simulink model "Control_test"  (R2014b)
settings: Solver=FixedStepDiscrete  StartTime=0.0  StopTime=Inf  FixedStep=0.001  RelTol=1e-3
PostLoadFcn:
  | , if any(exist('dsrtsu_mdlpostloadfcn', 'file') == [2, 3, 6]), try dsrtsu_mdlpostloadfcn('Execute', bdroot); catch fprintf('Error in PostLoadFcn (dsrtsu_mdlpostloadfcn) for model "%s":\n %s\n', bdroot, lasterr); end, end,
undefined symbols (not defined in the file or in its folder): dtLocal, slcm
libraries: rtican x163, simulink x14
(part 13 of 34)

== system Control_test/InputProcessing/CameraCanProcessing/Obstacle_Data_C_5 ==
  Bus Creator : BusCreator  Inputs=6
  Obstacle_Data_C_5 : rtican/RTICAN Receive (RX)   Reserved1=[]  Reserved2=[]  Reserved3=[]  Reserved4=[]  SfcnMessage=[]  Msg_Struct=[]  BoardTypeNo=[]  BoardNo=[]  ChannelNo=[]  Parameters=[]  DialogFcn=[]  UnitName=[]  Revision=[]  UnitValues=[]  DSProperties=struct('RTI',struct('Version',uint32(5),'BlockType',struct('isSLSource',uint8(1),'isSLSink',uint8(1),'isHWSource',uint8(0),'isHWSink',uint8(0),'isSetup',uint8(0),'isInline',uint8(1),'isNonInline',uint8(0),'isInterrupt',uint8(0),'isChannelwise',uint8(0)),'IOBoardType','RTICAN','UnitType','MESSAGE','Identifier','RX','DialogType','MSVC','BlockSet','RTICAN','SlaveProcessor','CAN'))  RTIBlockInterface=struct('OutputPortsWidth',int32([1 1 1 1 1 1]),'OutputPortsActive',[1 1 1 1 1 1],'OutputPortsName',{{'Alive_Counter_C_5','ObstacleWidth_C_5','ObjectMode_C_5','ObjectType_C_5','TTC_C_5','VisionScale_C_5'}},'OutputPortsDataType',{{'SS_DOUBLE','SS_DOUBLE','SS_DOUBLE','SS_DOUBLE','SS_DOUBLE','SS_DOUBLE'}},'OutputPortsLabel',{{'Alive_Counter_C_5','ObstacleWidth_C_5','ObjectMode_C_5','ObjectType_C_5','TTC_C_5','VisionScale_C_5'}},'OutputPortsLabelMode','ON','InputPortsWidth',int32(0),'InputPortsActive',0,'DialogFcn','rtican_message_interface_gui','BlockDisplay',{{'','center'}},'IconTransparency','on','ParameterTunableNames',{{}},'InitLevel',3,'BlockName',struct('Token',{{'Obstacle_Data_C_5'}}),'SampleTime',{{0.01}},'TriggerPort',{{'none'}},'EnablePort',{{'none'}})  RTIBlockParameters=struct('BoardTypeNo',{{1,'OFF',[]}},'BoardNo',{{1,'ON',[1 16]}},'ChannelNo',{{2,'ON',[1 2]}},'Parameters',{{struct('DataFileSupport',struct('DataFileSelectedMaster',1,'DataFileSelectedLocal',1,'DataFileName',['c:\users\mpc\desktop\hyundai car setup\rt2000_can_mod.dbc|c:\users\mpc\desktop\hyundai car setup\mobileye spec new\mobileye_mando_camera_ucb_v2.dbc|'],'DataFileDate',['18-Sep-2013 17:55:24'],'SelectedFile','..\..\dbcfiles\mobileye_mando_camera_ucb_v2.dbc','InterfaceFcn','rtican_dbc_file_parser'),'Options',struct('StatusSelected',0,'TimeSelected',0,'DeltaTimeSelected',0,'BytePortSelected',0,'MessageLengthSelected',0,'TriggerPort',struct('Selected',0,'TriggerType',0),'UserCoding',struct('Selected',0,'InterfaceFile','UserDecodingFile','FcnName','UserDecodeFcn','InportSelected',0,'InportWidth',1,'OutportSelected',0,'OutportWidth',1),'EnablePortSelected',0,'SignalOnPortnameSelected',1,'UseRXService',0),'Message',struct('MsgOnBlocknameSelected',1,'MsgName','Obstacle_Data_C_5','MsgIdFormat',0,'MsgId',1860,'MsgLength',6,'NumSignals',6,'SampleTime',0.01,'Signal',struct('SgnName',{'Alive_Counter_C_5','ObstacleWidth_C_5','ObjectMode_C_5','ObjectType_C_5','TTC_C_5','VisionScale_C_5'},'SgnStartBit',{0,8,16,18,22,32},'SgnLength',{2,8,2,4,10,12},'ByteLayout',{0,0,0,0,0,0},'Factor',{1,0.05,1,1,0.01,0.005},'Offset',{0,0,0,0,0,-8},'SgnComment',{'','','','','',''},'SgnUnit',{'','m','','','',''},'Min',{0,0,0,0,0,0},'Max',{0,0,0,0,0,0},'SgnType',{0,0,0,0,0,0},'SLDataType',{'SS_DOUBLE','SS_DOUBLE','SS_DOUBLE','SS_DOUBLE','SS_DOUBLE','SS_DOUBLE'},'DataType',{0,0,0,0,0,0},'ModeValue',{-1,-1,-1,-1,-1,-1}),'MsgIdNumFormat',0,'MsgComment',{{''}}),'Version',1.2,'general',struct('isFromLib',0)),'OFF',[]}},'GroupId',{{struct('Group',{{'RTICAN'}},'No',2,'Behavior',{{'NAMECHANGE'}},'BlockType',{{'SINK'}},'NameChangeFlag',0),'OFF',[]}},'SFcnRTICANMessage',{{struct('MsgType','RX','SFcnPortType','Scalar','MsgName','Obstacle_Data_C_5','MsgIdFormat','STD','MsgId',1860,'MsgLength',6,'NumSignals',6,'SampleTime',0.01,'Signal',struct('SgnName',{'Alive_Counter_C_5','ObstacleWidth_C_5','ObjectMode_C_5','ObjectType_C_5','TTC_C_5','VisionScale_C_5'},'SgnStartBit',{0,8,16,18,22,32},'SgnLength',{2,8,2,4,10,12},'ByteLayout',{['little endian'],['little endian'],['little endian'],['little endian'],['little endian'],['little endian']},'Factor',{1,0.05,1,1,0.01,0.005},'Offset',{0,0,0,0,0,-8},'SgnType',{'standard','standard','standard','standard','standard','standard'},'SLDataType',{'SS_DOUBLE','SS_DOUBLE','SS_DOUBLE','SS_DOUBLE','SS_DOUBLE','SS_DOUBLE'},'DataType',{['unsigned int'],['unsigned int'],['unsigned int'],['unsigned int'],['unsigned int'],['unsigned int']},'ModeValue',{-1,-1,-1,-1,-1,-1}),'StatusSelected','no','TimeSelected','no','DeltaTimeSelected','no','BytePortSelected','no','MessageLengthSelected','no','TriggerPort',struct('Selected','no','TriggerType',0),'UserCoding',struct('Selected','no','InterfaceFile','UserDecodingFile','FcnName','UserDecodeFcn','InportSelected','no','InportWidth',1,'OutportSelected','no','OutportWidth',1),'EnablePortSelected','no','UseRXService','no','BoardType','DS1','BoardNo',1,'ControllerNo',2),'OFF',[]}},'TLCFileName',{{'rtican_rx_message','OFF',[]}})  RTISFcnParameters=struct('SFcnRTICANMessage','struct','TLCFileName','char')  RTIBlockParaDefault=struct('BoardTypeNo',4302,'BoardNo',1,'ChannelNo',1,'Parameters',struct('DataFileSupport',struct('DataFileSelectedMaster',0,'DataFileSelectedLocal',0,'DataFileName','','DataFileDate','','SelectedFile',['<no file selected>']),'Options',struct('StatusSelected',1,'TimeSelected',1,'DeltaTimeSelected',1,'BytePortSelected',0,'MessageLengthSelected',0,'TriggerPort',struct('Selected',0,'TriggerType','rising'),'UserCoding',struct('Selected',0,'InterfaceFile','UserDecodingFile','FcnName','UserDecodeFcn','InportSelected',0,'InportWidth',1,'OutportSelected',0,'OutportWidth',1),'EnablePortSelected',0,'SignalOnPortnameSelected',1,'UseRXService',0),'Message',struct('MsgOnBlocknameSelected',0,'MsgName',['RX Message'],'MsgIdFormat',0,'MsgId',100,'MsgLength',8,'NumSignals',1,'SampleTime',-1,'Signal',struct('SgnName',['RX signal'],'SgnStartBit',0,'SgnLength',8,'SgnType',0,'ModeValue',-1,'DataType',0,'SLDataType','SS_DOUBLE','ByteLayout',0,'Factor',1,'Offset',0,'Min',0,'Max',255,'SgnComment',{{}},'SgnUnit',''),'MsgIdNumFormat',0,'MsgComment',{{''}}),'Version',1.2,'general',struct('isFromLib',1)),'GroupId',struct('Group',{{'RTICAN'}},'No',1,'Behavior',{{'NAMECHANGE'}},'BlockType',{{'SINK'}},'NameChangeFlag',0),'SFcnRTICANMessage',struct('MsgType','RX','MsgName',['RX Message'],'MsgIdFormat','STD','MsgId',100,'MsgLength',8,'NumSignals',1,'SampleTime',-1,'Signal',struct('SgnName',['RX signal'],'SgnStartBit',0,'SgnLength',8,'SgnType','standard','ModeValue',-1,'DataType',['unsigned int'],'ByteLayout',['little endian'],'SLDataType','SS_DOUBLE','Factor',1,'Offset',0),'StatusSelected','yes','TimeSelected','yes','DeltaTimeSelected','yes','BytePortSelected','no','MessageLengthSelected','no','EnablePortSelected','no','UserCoding',struct('Selected','no','InterfaceFile','UserDecodingFile','FcnName','UserDecodeFcn','InportSelected','no','InportWidth',1,'OutportSelected','no','OutportWidth',1),'TriggerPort',struct('Selected','no','TriggerType','rising'),'UseRXService','no','BoardType','DS4302','BoardNo',1,'ControllerNo',1,'SFcnPortType','Scalar'),'TLCFileName','rtican_rx_message')
      settings: AttributesFormatString=Group Id: RTICAN2\n
  Obstacle_Data_C_5_CAN : Outport
  wires:
  Bus Creator/1 -> Obstacle_Data_C_5_CAN/1
  Obstacle_Data_C_5/1 -> Bus Creator/1  "Alive_Counter_C_5"
  Obstacle_Data_C_5/2 -> Bus Creator/2  "ObstacleWidth_C_5"
  Obstacle_Data_C_5/3 -> Bus Creator/3  "ObjectMode_C_5"
  Obstacle_Data_C_5/4 -> Bus Creator/4  "ObjectType_C_5"
  Obstacle_Data_C_5/5 -> Bus Creator/5  "TTC_C_5"
  Obstacle_Data_C_5/6 -> Bus Creator/6  "VisionScale_C_5"

== system Control_test/InputProcessing/CameraCanProcessing/Obstacle_Data_C_6 ==
  Bus Creator : BusCreator  Inputs=6
  Obstacle_Data_C_6 : rtican/RTICAN Receive (RX)   Reserved1=[]  Reserved2=[]  Reserved3=[]  Reserved4=[]  SfcnMessage=[]  Msg_Struct=[]  BoardTypeNo=[]  BoardNo=[]  ChannelNo=[]  Parameters=[]  DialogFcn=[]  UnitName=[]  Revision=[]  UnitValues=[]  DSProperties=struct('RTI',struct('Version',uint32(5),'BlockType',struct('isSLSource',uint8(1),'isSLSink',uint8(1),'isHWSource',uint8(0),'isHWSink',uint8(0),'isSetup',uint8(0),'isInline',uint8(1),'isNonInline',uint8(0),'isInterrupt',uint8(0),'isChannelwise',uint8(0)),'IOBoardType','RTICAN','UnitType','MESSAGE','Identifier','RX','DialogType','MSVC','BlockSet','RTICAN','SlaveProcessor','CAN'))  RTIBlockInterface=struct('OutputPortsWidth',int32([1 1 1 1 1 1]),'OutputPortsActive',[1 1 1 1 1 1],'OutputPortsName',{{'Alive_Counter_C_6','ObstacleWidth_C_6','ObjectMode_C_6','ObjectType_C_6','TTC_C_6','VisionScale_C_6'}},'OutputPortsDataType',{{'SS_DOUBLE','SS_DOUBLE','SS_DOUBLE','SS_DOUBLE','SS_DOUBLE','SS_DOUBLE'}},'OutputPortsLabel',{{'Alive_Counter_C_6','ObstacleWidth_C_6','ObjectMode_C_6','ObjectType_C_6','TTC_C_6','VisionScale_C_6'}},'OutputPortsLabelMode','ON','InputPortsWidth',int32(0),'InputPortsActive',0,'DialogFcn','rtican_message_interface_gui','BlockDisplay',{{'','center'}},'IconTransparency','on','ParameterTunableNames',{{}},'InitLevel',3,'BlockName',struct('Token',{{'Obstacle_Data_C_6'}}),'SampleTime',{{0.01}},'TriggerPort',{{'none'}},'EnablePort',{{'none'}})  RTIBlockParameters=struct('BoardTypeNo',{{1,'OFF',[]}},'BoardNo',{{1,'ON',[1 16]}},'ChannelNo',{{2,'ON',[1 2]}},'Parameters',{{struct('DataFileSupport',struct('DataFileSelectedMaster',1,'DataFileSelectedLocal',1,'DataFileName',['c:\users\mpc\desktop\hyundai car setup\rt2000_can_mod.dbc|c:\users\mpc\desktop\hyundai car setup\mobileye spec new\mobileye_mando_camera_ucb_v2.dbc|'],'DataFileDate',['18-Sep-2013 17:55:24'],'SelectedFile','..\..\dbcfiles\mobileye_mando_camera_ucb_v2.dbc','InterfaceFcn','rtican_dbc_file_parser'),'Options',struct('StatusSelected',0,'TimeSelected',0,'DeltaTimeSelected',0,'BytePortSelected',0,'MessageLengthSelected',0,'TriggerPort',struct('Selected',0,'TriggerType',0),'UserCoding',struct('Selected',0,'InterfaceFile','UserDecodingFile','FcnName','UserDecodeFcn','InportSelected',0,'InportWidth',1,'OutportSelected',0,'OutportWidth',1),'EnablePortSelected',0,'SignalOnPortnameSelected',1,'UseRXService',0),'Message',struct('MsgOnBlocknameSelected',1,'MsgName','Obstacle_Data_C_6','MsgIdFormat',0,'MsgId',1863,'MsgLength',6,'NumSignals',6,'SampleTime',0.01,'Signal',struct('SgnName',{'Alive_Counter_C_6','ObstacleWidth_C_6','ObjectMode_C_6','ObjectType_C_6','TTC_C_6','VisionScale_C_6'},'SgnStartBit',{0,8,16,18,22,32},'SgnLength',{2,8,2,4,10,12},'ByteLayout',{0,0,0,0,0,0},'Factor',{1,0.05,1,1,0.01,0.005},'Offset',{0,0,0,0,0,-8},'SgnComment',{'','','','','',''},'SgnUnit',{'','m','','','',''},'Min',{0,0,0,0,0,0},'Max',{0,0,0,0,0,0},'SgnType',{0,0,0,0,0,0},'SLDataType',{'SS_DOUBLE','SS_DOUBLE','SS_DOUBLE','SS_DOUBLE','SS_DOUBLE','SS_DOUBLE'},'DataType',{0,0,0,0,0,0},'ModeValue',{-1,-1,-1,-1,-1,-1}),'MsgIdNumFormat',0,'MsgComment',{{''}}),'Version',1.2,'general',struct('isFromLib',0)),'OFF',[]}},'GroupId',{{struct('Group',{{'RTICAN'}},'No',2,'Behavior',{{'NAMECHANGE'}},'BlockType',{{'SINK'}},'NameChangeFlag',0),'OFF',[]}},'SFcnRTICANMessage',{{struct('MsgType','RX','SFcnPortType','Scalar','MsgName','Obstacle_Data_C_6','MsgIdFormat','STD','MsgId',1863,'MsgLength',6,'NumSignals',6,'SampleTime',0.01,'Signal',struct('SgnName',{'Alive_Counter_C_6','ObstacleWidth_C_6','ObjectMode_C_6','ObjectType_C_6','TTC_C_6','VisionScale_C_6'},'SgnStartBit',{0,8,16,18,22,32},'SgnLength',{2,8,2,4,10,12},'ByteLayout',{['little endian'],['little endian'],['little endian'],['little endian'],['little endian'],['little endian']},'Factor',{1,0.05,1,1,0.01,0.005},'Offset',{0,0,0,0,0,-8},'SgnType',{'standard','standard','standard','standard','standard','standard'},'SLDataType',{'SS_DOUBLE','SS_DOUBLE','SS_DOUBLE','SS_DOUBLE','SS_DOUBLE','SS_DOUBLE'},'DataType',{['unsigned int'],['unsigned int'],['unsigned int'],['unsigned int'],['unsigned int'],['unsigned int']},'ModeValue',{-1,-1,-1,-1,-1,-1}),'StatusSelected','no','TimeSelected','no','DeltaTimeSelected','no','BytePortSelected','no','MessageLengthSelected','no','TriggerPort',struct('Selected','no','TriggerType',0),'UserCoding',struct('Selected','no','InterfaceFile','UserDecodingFile','FcnName','UserDecodeFcn','InportSelected','no','InportWidth',1,'OutportSelected','no','OutportWidth',1),'EnablePortSelected','no','UseRXService','no','BoardType','DS1','BoardNo',1,'ControllerNo',2),'OFF',[]}},'TLCFileName',{{'rtican_rx_message','OFF',[]}})  RTISFcnParameters=struct('SFcnRTICANMessage','struct','TLCFileName','char')  RTIBlockParaDefault=struct('BoardTypeNo',4302,'BoardNo',1,'ChannelNo',1,'Parameters',struct('DataFileSupport',struct('DataFileSelectedMaster',0,'DataFileSelectedLocal',0,'DataFileName','','DataFileDate','','SelectedFile',['<no file selected>']),'Options',struct('StatusSelected',1,'TimeSelected',1,'DeltaTimeSelected',1,'BytePortSelected',0,'MessageLengthSelected',0,'TriggerPort',struct('Selected',0,'TriggerType','rising'),'UserCoding',struct('Selected',0,'InterfaceFile','UserDecodingFile','FcnName','UserDecodeFcn','InportSelected',0,'InportWidth',1,'OutportSelected',0,'OutportWidth',1),'EnablePortSelected',0,'SignalOnPortnameSelected',1,'UseRXService',0),'Message',struct('MsgOnBlocknameSelected',0,'MsgName',['RX Message'],'MsgIdFormat',0,'MsgId',100,'MsgLength',8,'NumSignals',1,'SampleTime',-1,'Signal',struct('SgnName',['RX signal'],'SgnStartBit',0,'SgnLength',8,'SgnType',0,'ModeValue',-1,'DataType',0,'SLDataType','SS_DOUBLE','ByteLayout',0,'Factor',1,'Offset',0,'Min',0,'Max',255,'SgnComment',{{}},'SgnUnit',''),'MsgIdNumFormat',0,'MsgComment',{{''}}),'Version',1.2,'general',struct('isFromLib',1)),'GroupId',struct('Group',{{'RTICAN'}},'No',1,'Behavior',{{'NAMECHANGE'}},'BlockType',{{'SINK'}},'NameChangeFlag',0),'SFcnRTICANMessage',struct('MsgType','RX','MsgName',['RX Message'],'MsgIdFormat','STD','MsgId',100,'MsgLength',8,'NumSignals',1,'SampleTime',-1,'Signal',struct('SgnName',['RX signal'],'SgnStartBit',0,'SgnLength',8,'SgnType','standard','ModeValue',-1,'DataType',['unsigned int'],'ByteLayout',['little endian'],'SLDataType','SS_DOUBLE','Factor',1,'Offset',0),'StatusSelected','yes','TimeSelected','yes','DeltaTimeSelected','yes','BytePortSelected','no','MessageLengthSelected','no','EnablePortSelected','no','UserCoding',struct('Selected','no','InterfaceFile','UserDecodingFile','FcnName','UserDecodeFcn','InportSelected','no','InportWidth',1,'OutportSelected','no','OutportWidth',1),'TriggerPort',struct('Selected','no','TriggerType','rising'),'UseRXService','no','BoardType','DS4302','BoardNo',1,'ControllerNo',1,'SFcnPortType','Scalar'),'TLCFileName','rtican_rx_message')
      settings: AttributesFormatString=Group Id: RTICAN2\n
  Obstacle_Data_C_6_CAN : Outport
  wires:
  Bus Creator/1 -> Obstacle_Data_C_6_CAN/1
  Obstacle_Data_C_6/1 -> Bus Creator/1  "Alive_Counter_C_6"
  Obstacle_Data_C_6/2 -> Bus Creator/2  "ObstacleWidth_C_6"
  Obstacle_Data_C_6/3 -> Bus Creator/3  "ObjectMode_C_6"
  Obstacle_Data_C_6/4 -> Bus Creator/4  "ObjectType_C_6"
  Obstacle_Data_C_6/5 -> Bus Creator/5  "TTC_C_6"
  Obstacle_Data_C_6/6 -> Bus Creator/6  "VisionScale_C_6"

== system Control_test/InputProcessing/CameraCanProcessing/Obstacle_Data_C_7 ==
  Bus Creator : BusCreator  Inputs=6
  Obstacle_Data_C_7 : rtican/RTICAN Receive (RX)   Reserved1=[]  Reserved2=[]  Reserved3=[]  Reserved4=[]  SfcnMessage=[]  Msg_Struct=[]  BoardTypeNo=[]  BoardNo=[]  ChannelNo=[]  Parameters=[]  DialogFcn=[]  UnitName=[]  Revision=[]  UnitValues=[]  DSProperties=struct('RTI',struct('Version',uint32(5),'BlockType',struct('isSLSource',uint8(1),'isSLSink',uint8(1),'isHWSource',uint8(0),'isHWSink',uint8(0),'isSetup',uint8(0),'isInline',uint8(1),'isNonInline',uint8(0),'isInterrupt',uint8(0),'isChannelwise',uint8(0)),'IOBoardType','RTICAN','UnitType','MESSAGE','Identifier','RX','DialogType','MSVC','BlockSet','RTICAN','SlaveProcessor','CAN'))  RTIBlockInterface=struct('OutputPortsWidth',int32([1 1 1 1 1 1]),'OutputPortsActive',[1 1 1 1 1 1],'OutputPortsName',{{'Alive_Counter_C_7','ObstacleWidth_C_7','ObjectMode_C_7','ObjectType_C_7','TTC_C_7','VisionScale_C_7'}},'OutputPortsDataType',{{'SS_DOUBLE','SS_DOUBLE','SS_DOUBLE','SS_DOUBLE','SS_DOUBLE','SS_DOUBLE'}},'OutputPortsLabel',{{'Alive_Counter_C_7','ObstacleWidth_C_7','ObjectMode_C_7','ObjectType_C_7','TTC_C_7','VisionScale_C_7'}},'OutputPortsLabelMode','ON','InputPortsWidth',int32(0),'InputPortsActive',0,'DialogFcn','rtican_message_interface_gui','BlockDisplay',{{'','center'}},'IconTransparency','on','ParameterTunableNames',{{}},'InitLevel',3,'BlockName',struct('Token',{{'Obstacle_Data_C_7'}}),'SampleTime',{{0.01}},'TriggerPort',{{'none'}},'EnablePort',{{'none'}})  RTIBlockParameters=struct('BoardTypeNo',{{1,'OFF',[]}},'BoardNo',{{1,'ON',[1 16]}},'ChannelNo',{{2,'ON',[1 2]}},'Parameters',{{struct('DataFileSupport',struct('DataFileSelectedMaster',1,'DataFileSelectedLocal',1,'DataFileName',['c:\users\mpc\desktop\hyundai car setup\rt2000_can_mod.dbc|c:\users\mpc\desktop\hyundai car setup\mobileye spec new\mobileye_mando_camera_ucb_v2.dbc|'],'DataFileDate',['18-Sep-2013 17:55:24'],'SelectedFile','..\..\dbcfiles\mobileye_mando_camera_ucb_v2.dbc','InterfaceFcn','rtican_dbc_file_parser'),'Options',struct('StatusSelected',0,'TimeSelected',0,'DeltaTimeSelected',0,'BytePortSelected',0,'MessageLengthSelected',0,'TriggerPort',struct('Selected',0,'TriggerType',0),'UserCoding',struct('Selected',0,'InterfaceFile','UserDecodingFile','FcnName','UserDecodeFcn','InportSelected',0,'InportWidth',1,'OutportSelected',0,'OutportWidth',1),'EnablePortSelected',0,'SignalOnPortnameSelected',1,'UseRXService',0),'Message',struct('MsgOnBlocknameSelected',1,'MsgName','Obstacle_Data_C_7','MsgIdFormat',0,'MsgId',1866,'MsgLength',6,'NumSignals',6,'SampleTime',0.01,'Signal',struct('SgnName',{'Alive_Counter_C_7','ObstacleWidth_C_7','ObjectMode_C_7','ObjectType_C_7','TTC_C_7','VisionScale_C_7'},'SgnStartBit',{0,8,16,18,22,32},'SgnLength',{2,8,2,4,10,12},'ByteLayout',{0,0,0,0,0,0},'Factor',{1,0.05,1,1,0.01,0.005},'Offset',{0,0,0,0,0,-8},'SgnComment',{'','','','','',''},'SgnUnit',{'','m','','','',''},'Min',{0,0,0,0,0,0},'Max',{0,0,0,0,0,0},'SgnType',{0,0,0,0,0,0},'SLDataType',{'SS_DOUBLE','SS_DOUBLE','SS_DOUBLE','SS_DOUBLE','SS_DOUBLE','SS_DOUBLE'},'DataType',{0,0,0,0,0,0},'ModeValue',{-1,-1,-1,-1,-1,-1}),'MsgIdNumFormat',0,'MsgComment',{{''}}),'Version',1.2,'general',struct('isFromLib',0)),'OFF',[]}},'GroupId',{{struct('Group',{{'RTICAN'}},'No',2,'Behavior',{{'NAMECHANGE'}},'BlockType',{{'SINK'}},'NameChangeFlag',0),'OFF',[]}},'SFcnRTICANMessage',{{struct('MsgType','RX','SFcnPortType','Scalar','MsgName','Obstacle_Data_C_7','MsgIdFormat','STD','MsgId',1866,'MsgLength',6,'NumSignals',6,'SampleTime',0.01,'Signal',struct('SgnName',{'Alive_Counter_C_7','ObstacleWidth_C_7','ObjectMode_C_7','ObjectType_C_7','TTC_C_7','VisionScale_C_7'},'SgnStartBit',{0,8,16,18,22,32},'SgnLength',{2,8,2,4,10,12},'ByteLayout',{['little endian'],['little endian'],['little endian'],['little endian'],['little endian'],['little endian']},'Factor',{1,0.05,1,1,0.01,0.005},'Offset',{0,0,0,0,0,-8},'SgnType',{'standard','standard','standard','standard','standard','standard'},'SLDataType',{'SS_DOUBLE','SS_DOUBLE','SS_DOUBLE','SS_DOUBLE','SS_DOUBLE','SS_DOUBLE'},'DataType',{['unsigned int'],['unsigned int'],['unsigned int'],['unsigned int'],['unsigned int'],['unsigned int']},'ModeValue',{-1,-1,-1,-1,-1,-1}),'StatusSelected','no','TimeSelected','no','DeltaTimeSelected','no','BytePortSelected','no','MessageLengthSelected','no','TriggerPort',struct('Selected','no','TriggerType',0),'UserCoding',struct('Selected','no','InterfaceFile','UserDecodingFile','FcnName','UserDecodeFcn','InportSelected','no','InportWidth',1,'OutportSelected','no','OutportWidth',1),'EnablePortSelected','no','UseRXService','no','BoardType','DS1','BoardNo',1,'ControllerNo',2),'OFF',[]}},'TLCFileName',{{'rtican_rx_message','OFF',[]}})  RTISFcnParameters=struct('SFcnRTICANMessage','struct','TLCFileName','char')  RTIBlockParaDefault=struct('BoardTypeNo',4302,'BoardNo',1,'ChannelNo',1,'Parameters',struct('DataFileSupport',struct('DataFileSelectedMaster',0,'DataFileSelectedLocal',0,'DataFileName','','DataFileDate','','SelectedFile',['<no file selected>']),'Options',struct('StatusSelected',1,'TimeSelected',1,'DeltaTimeSelected',1,'BytePortSelected',0,'MessageLengthSelected',0,'TriggerPort',struct('Selected',0,'TriggerType','rising'),'UserCoding',struct('Selected',0,'InterfaceFile','UserDecodingFile','FcnName','UserDecodeFcn','InportSelected',0,'InportWidth',1,'OutportSelected',0,'OutportWidth',1),'EnablePortSelected',0,'SignalOnPortnameSelected',1,'UseRXService',0),'Message',struct('MsgOnBlocknameSelected',0,'MsgName',['RX Message'],'MsgIdFormat',0,'MsgId',100,'MsgLength',8,'NumSignals',1,'SampleTime',-1,'Signal',struct('SgnName',['RX signal'],'SgnStartBit',0,'SgnLength',8,'SgnType',0,'ModeValue',-1,'DataType',0,'SLDataType','SS_DOUBLE','ByteLayout',0,'Factor',1,'Offset',0,'Min',0,'Max',255,'SgnComment',{{}},'SgnUnit',''),'MsgIdNumFormat',0,'MsgComment',{{''}}),'Version',1.2,'general',struct('isFromLib',1)),'GroupId',struct('Group',{{'RTICAN'}},'No',1,'Behavior',{{'NAMECHANGE'}},'BlockType',{{'SINK'}},'NameChangeFlag',0),'SFcnRTICANMessage',struct('MsgType','RX','MsgName',['RX Message'],'MsgIdFormat','STD','MsgId',100,'MsgLength',8,'NumSignals',1,'SampleTime',-1,'Signal',struct('SgnName',['RX signal'],'SgnStartBit',0,'SgnLength',8,'SgnType','standard','ModeValue',-1,'DataType',['unsigned int'],'ByteLayout',['little endian'],'SLDataType','SS_DOUBLE','Factor',1,'Offset',0),'StatusSelected','yes','TimeSelected','yes','DeltaTimeSelected','yes','BytePortSelected','no','MessageLengthSelected','no','EnablePortSelected','no','UserCoding',struct('Selected','no','InterfaceFile','UserDecodingFile','FcnName','UserDecodeFcn','InportSelected','no','InportWidth',1,'OutportSelected','no','OutportWidth',1),'TriggerPort',struct('Selected','no','TriggerType','rising'),'UseRXService','no','BoardType','DS4302','BoardNo',1,'ControllerNo',1,'SFcnPortType','Scalar'),'TLCFileName','rtican_rx_message')
      settings: AttributesFormatString=Group Id: RTICAN2\n
  Obstacle_Data_C_7_CAN : Outport
  wires:
  Bus Creator/1 -> Obstacle_Data_C_7_CAN/1
  Obstacle_Data_C_7/1 -> Bus Creator/1  "Alive_Counter_C_7"
  Obstacle_Data_C_7/2 -> Bus Creator/2  "ObstacleWidth_C_7"
  Obstacle_Data_C_7/3 -> Bus Creator/3  "ObjectMode_C_7"
  Obstacle_Data_C_7/4 -> Bus Creator/4  "ObjectType_C_7"
  Obstacle_Data_C_7/5 -> Bus Creator/5  "TTC_C_7"
  Obstacle_Data_C_7/6 -> Bus Creator/6  "VisionScale_C_7"

== system Control_test/InputProcessing/CameraCanProcessing/Obstacle_Data_C_8 ==
  Bus Creator : BusCreator  Inputs=6
  Obstacle_Data_C_8 : rtican/RTICAN Receive (RX)   Reserved1=[]  Reserved2=[]  Reserved3=[]  Reserved4=[]  SfcnMessage=[]  Msg_Struct=[]  BoardTypeNo=[]  BoardNo=[]  ChannelNo=[]  Parameters=[]  DialogFcn=[]  UnitName=[]  Revision=[]  UnitValues=[]  DSProperties=struct('RTI',struct('Version',uint32(5),'BlockType',struct('isSLSource',uint8(1),'isSLSink',uint8(1),'isHWSource',uint8(0),'isHWSink',uint8(0),'isSetup',uint8(0),'isInline',uint8(1),'isNonInline',uint8(0),'isInterrupt',uint8(0),'isChannelwise',uint8(0)),'IOBoardType','RTICAN','UnitType','MESSAGE','Identifier','RX','DialogType','MSVC','BlockSet','RTICAN','SlaveProcessor','CAN'))  RTIBlockInterface=struct('OutputPortsWidth',int32([1 1 1 1 1 1]),'OutputPortsActive',[1 1 1 1 1 1],'OutputPortsName',{{'Alive_Counter_C_8','ObstacleWidth_C_8','ObjectMode_C_8','ObjectType_C_8','TTC_C_8','VisionScale_C_8'}},'OutputPortsDataType',{{'SS_DOUBLE','SS_DOUBLE','SS_DOUBLE','SS_DOUBLE','SS_DOUBLE','SS_DOUBLE'}},'OutputPortsLabel',{{'Alive_Counter_C_8','ObstacleWidth_C_8','ObjectMode_C_8','ObjectType_C_8','TTC_C_8','VisionScale_C_8'}},'OutputPortsLabelMode','ON','InputPortsWidth',int32(0),'InputPortsActive',0,'DialogFcn','rtican_message_interface_gui','BlockDisplay',{{'','center'}},'IconTransparency','on','ParameterTunableNames',{{}},'InitLevel',3,'BlockName',struct('Token',{{'Obstacle_Data_C_8'}}),'SampleTime',{{0.01}},'TriggerPort',{{'none'}},'EnablePort',{{'none'}})  RTIBlockParameters=struct('BoardTypeNo',{{1,'OFF',[]}},'BoardNo',{{1,'ON',[1 16]}},'ChannelNo',{{2,'ON',[1 2]}},'Parameters',{{struct('DataFileSupport',struct('DataFileSelectedMaster',1,'DataFileSelectedLocal',1,'DataFileName',['c:\users\mpc\desktop\hyundai car setup\rt2000_can_mod.dbc|c:\users\mpc\desktop\hyundai car setup\mobileye spec new\mobileye_mando_camera_ucb_v2.dbc|'],'DataFileDate',['18-Sep-2013 17:55:24'],'SelectedFile','..\..\dbcfiles\mobileye_mando_camera_ucb_v2.dbc','InterfaceFcn','rtican_dbc_file_parser'),'Options',struct('StatusSelected',0,'TimeSelected',0,'DeltaTimeSelected',0,'BytePortSelected',0,'MessageLengthSelected',0,'TriggerPort',struct('Selected',0,'TriggerType',0),'UserCoding',struct('Selected',0,'InterfaceFile','UserDecodingFile','FcnName','UserDecodeFcn','InportSelected',0,'InportWidth',1,'OutportSelected',0,'OutportWidth',1),'EnablePortSelected',0,'SignalOnPortnameSelected',1,'UseRXService',0),'Message',struct('MsgOnBlocknameSelected',1,'MsgName','Obstacle_Data_C_8','MsgIdFormat',0,'MsgId',1869,'MsgLength',6,'NumSignals',6,'SampleTime',0.01,'Signal',struct('SgnName',{'Alive_Counter_C_8','ObstacleWidth_C_8','ObjectMode_C_8','ObjectType_C_8','TTC_C_8','VisionScale_C_8'},'SgnStartBit',{0,8,16,18,22,32},'SgnLength',{2,8,2,4,10,12},'ByteLayout',{0,0,0,0,0,0},'Factor',{1,0.05,1,1,0.01,0.005},'Offset',{0,0,0,0,0,-8},'SgnComment',{'','','','','',''},'SgnUnit',{'','m','','','',''},'Min',{0,0,0,0,0,0},'Max',{0,0,0,0,0,0},'SgnType',{0,0,0,0,0,0},'SLDataType',{'SS_DOUBLE','SS_DOUBLE','SS_DOUBLE','SS_DOUBLE','SS_DOUBLE','SS_DOUBLE'},'DataType',{0,0,0,0,0,0},'ModeValue',{-1,-1,-1,-1,-1,-1}),'MsgIdNumFormat',0,'MsgComment',{{''}}),'Version',1.2,'general',struct('isFromLib',0)),'OFF',[]}},'GroupId',{{struct('Group',{{'RTICAN'}},'No',2,'Behavior',{{'NAMECHANGE'}},'BlockType',{{'SINK'}},'NameChangeFlag',0),'OFF',[]}},'SFcnRTICANMessage',{{struct('MsgType','RX','SFcnPortType','Scalar','MsgName','Obstacle_Data_C_8','MsgIdFormat','STD','MsgId',1869,'MsgLength',6,'NumSignals',6,'SampleTime',0.01,'Signal',struct('SgnName',{'Alive_Counter_C_8','ObstacleWidth_C_8','ObjectMode_C_8','ObjectType_C_8','TTC_C_8','VisionScale_C_8'},'SgnStartBit',{0,8,16,18,22,32},'SgnLength',{2,8,2,4,10,12},'ByteLayout',{['little endian'],['little endian'],['little endian'],['little endian'],['little endian'],['little endian']},'Factor',{1,0.05,1,1,0.01,0.005},'Offset',{0,0,0,0,0,-8},'SgnType',{'standard','standard','standard','standard','standard','standard'},'SLDataType',{'SS_DOUBLE','SS_DOUBLE','SS_DOUBLE','SS_DOUBLE','SS_DOUBLE','SS_DOUBLE'},'DataType',{['unsigned int'],['unsigned int'],['unsigned int'],['unsigned int'],['unsigned int'],['unsigned int']},'ModeValue',{-1,-1,-1,-1,-1,-1}),'StatusSelected','no','TimeSelected','no','DeltaTimeSelected','no','BytePortSelected','no','MessageLengthSelected','no','TriggerPort',struct('Selected','no','TriggerType',0),'UserCoding',struct('Selected','no','InterfaceFile','UserDecodingFile','FcnName','UserDecodeFcn','InportSelected','no','InportWidth',1,'OutportSelected','no','OutportWidth',1),'EnablePortSelected','no','UseRXService','no','BoardType','DS1','BoardNo',1,'ControllerNo',2),'OFF',[]}},'TLCFileName',{{'rtican_rx_message','OFF',[]}})  RTISFcnParameters=struct('SFcnRTICANMessage','struct','TLCFileName','char')  RTIBlockParaDefault=struct('BoardTypeNo',4302,'BoardNo',1,'ChannelNo',1,'Parameters',struct('DataFileSupport',struct('DataFileSelectedMaster',0,'DataFileSelectedLocal',0,'DataFileName','','DataFileDate','','SelectedFile',['<no file selected>']),'Options',struct('StatusSelected',1,'TimeSelected',1,'DeltaTimeSelected',1,'BytePortSelected',0,'MessageLengthSelected',0,'TriggerPort',struct('Selected',0,'TriggerType','rising'),'UserCoding',struct('Selected',0,'InterfaceFile','UserDecodingFile','FcnName','UserDecodeFcn','InportSelected',0,'InportWidth',1,'OutportSelected',0,'OutportWidth',1),'EnablePortSelected',0,'SignalOnPortnameSelected',1,'UseRXService',0),'Message',struct('MsgOnBlocknameSelected',0,'MsgName',['RX Message'],'MsgIdFormat',0,'MsgId',100,'MsgLength',8,'NumSignals',1,'SampleTime',-1,'Signal',struct('SgnName',['RX signal'],'SgnStartBit',0,'SgnLength',8,'SgnType',0,'ModeValue',-1,'DataType',0,'SLDataType','SS_DOUBLE','ByteLayout',0,'Factor',1,'Offset',0,'Min',0,'Max',255,'SgnComment',{{}},'SgnUnit',''),'MsgIdNumFormat',0,'MsgComment',{{''}}),'Version',1.2,'general',struct('isFromLib',1)),'GroupId',struct('Group',{{'RTICAN'}},'No',1,'Behavior',{{'NAMECHANGE'}},'BlockType',{{'SINK'}},'NameChangeFlag',0),'SFcnRTICANMessage',struct('MsgType','RX','MsgName',['RX Message'],'MsgIdFormat','STD','MsgId',100,'MsgLength',8,'NumSignals',1,'SampleTime',-1,'Signal',struct('SgnName',['RX signal'],'SgnStartBit',0,'SgnLength',8,'SgnType','standard','ModeValue',-1,'DataType',['unsigned int'],'ByteLayout',['little endian'],'SLDataType','SS_DOUBLE','Factor',1,'Offset',0),'StatusSelected','yes','TimeSelected','yes','DeltaTimeSelected','yes','BytePortSelected','no','MessageLengthSelected','no','EnablePortSelected','no','UserCoding',struct('Selected','no','InterfaceFile','UserDecodingFile','FcnName','UserDecodeFcn','InportSelected','no','InportWidth',1,'OutportSelected','no','OutportWidth',1),'TriggerPort',struct('Selected','no','TriggerType','rising'),'UseRXService','no','BoardType','DS4302','BoardNo',1,'ControllerNo',1,'SFcnPortType','Scalar'),'TLCFileName','rtican_rx_message')
      settings: AttributesFormatString=Group Id: RTICAN2\n
  Obstacle_Data_C_8_CAN : Outport
  wires:
  Bus Creator/1 -> Obstacle_Data_C_8_CAN/1
  Obstacle_Data_C_8/1 -> Bus Creator/1  "Alive_Counter_C_8"
  Obstacle_Data_C_8/2 -> Bus Creator/2  "ObstacleWidth_C_8"
  Obstacle_Data_C_8/3 -> Bus Creator/3  "ObjectMode_C_8"
  Obstacle_Data_C_8/4 -> Bus Creator/4  "ObjectType_C_8"
  Obstacle_Data_C_8/5 -> Bus Creator/5  "TTC_C_8"
  Obstacle_Data_C_8/6 -> Bus Creator/6  "VisionScale_C_8"

== system Control_test/InputProcessing/IBEOCANProcessing/IBEOESP2Processing ==
  In1 : Inport
  Bus Creator : BusCreator  Inputs=12
  Bus Selector3 : BusSelector  OutputSignals=LAT_ACCEL,LAT_ACCEL_STAT,LAT_ACCEL_DIAG,LONG_ACCEL,LONG_ACCEL_STAT,LONG_ACCEL_DIAG,CYL_PRES,CYL_PRES_STAT,CYL_PRESS_DIAG,YAW_RATE,YAW_RATE_STAT,YAW_RATE_DIAG
  ESP2 Processing : Subsystem
  Out1 : Outport
  wires:
  Bus Selector3/1 -> ESP2 Processing/1(LAT_ACCEL_CAN)  "<LAT_ACCEL>"
  Bus Selector3/2 -> ESP2 Processing/2(LAT_ACCEL_STAT_CAN)  "<LAT_ACCEL_STAT>"
  Bus Selector3/3 -> ESP2 Processing/3(LAT_ACCEL_DIAG_CAN)  "<LAT_ACCEL_DIAG>"
  Bus Selector3/4 -> ESP2 Processing/4(LONG_ACCEL_CAN)  "<LONG_ACCEL>"
  Bus Selector3/5 -> ESP2 Processing/5(LONG_ACCEL_STAT_CAN)  "<LONG_ACCEL_STAT>"
  Bus Selector3/6 -> ESP2 Processing/6(LONG_ACCEL_DIAG_CAN)  "<LONG_ACCEL_DIAG>"
  Bus Selector3/7 -> ESP2 Processing/7(CYL_PRES_CAN)  "<CYL_PRES>"
  Bus Selector3/8 -> ESP2 Processing/8(CYL_PRES_STAT_CAN)  "<CYL_PRES_STAT>"
  Bus Selector3/9 -> ESP2 Processing/9(CYL_PRES_DIAG_CAN)  "<CYL_PRESS_DIAG>"
  Bus Selector3/10 -> ESP2 Processing/10(YAW_RATE_CAN)  "<YAW_RATE>"
  Bus Selector3/11 -> ESP2 Processing/11(YAW_RATE_STAT_CAN)  "<YAW_RATE_STAT>"
  Bus Selector3/12 -> ESP2 Processing/12(YAW_RATE_DIAG_CAN)  "<YAW_RATE_DIAG>"
  ESP2 Processing/1(ipLatAccel [m/s2]) -> Bus Creator/1
  ESP2 Processing/2(ipLatAccelFail) -> Bus Creator/2
  ESP2 Processing/3(ipLatAccelDiag) -> Bus Creator/3
  ESP2 Processing/4(ipLongAccel [m/s2]) -> Bus Creator/4
  ESP2 Processing/5(ipLongAccelFail) -> Bus Creator/5
  ESP2 Processing/6(ipLongAccelDiag) -> Bus Creator/6
  ESP2 Processing/7(ipMsCylPress [bar]) -> Bus Creator/7
  ESP2 Processing/8(ipMsCylPressFail) -> Bus Creator/8
  ESP2 Processing/9(ipMsCylPressDiag) -> Bus Creator/9
  ESP2 Processing/10(ipYawRate [deg/s]) -> Bus Creator/10
  ESP2 Processing/11(ipYawRateFail) -> Bus Creator/11
  ESP2 Processing/12(ipYawRateDiag) -> Bus Creator/12
  Bus Creator/1 -> Out1/1  "ESP2DataCAN3"
  In1/1 -> Bus Selector3/1

== system Control_test/InputProcessing/IBEOCANProcessing/IBEOSASProcessing ==
  In1 : Inport
  Bus Creator4 : BusCreator  Inputs=6
  Bus Selector4 : BusSelector  OutputSignals=SAS_Angle,SAS_Speed,MsgCount,CheckSum
  SAS1 Processing : Subsystem
  Out1 : Outport
  wires:
  Bus Selector4/1 -> SAS1 Processing/1(SAS_Angle_CAN)  "<SAS_Angle>"
  Bus Selector4/2 -> SAS1 Processing/2(SAS_Speed_CAN)  "<SAS_Speed>"
  Bus Selector4/3 -> SAS1 Processing/3(MsgCount_CAN)  "<MsgCount>"
  Bus Selector4/4 -> SAS1 Processing/4(CheckSum_CAN)  "<CheckSum>"
  SAS1 Processing/1(ipStrAng [deg]) -> Bus Creator4/1
  SAS1 Processing/2(ipStrAngEr) -> Bus Creator4/2
  SAS1 Processing/3(ipStrSpd [deg/s]) -> Bus Creator4/3
  SAS1 Processing/4(ipStrSpdEr) -> Bus Creator4/4
  SAS1 Processing/5(ipSasCnt) -> Bus Creator4/5
  SAS1 Processing/6(ipSasCksum) -> Bus Creator4/6
  Bus Creator4/1 -> Out1/1  "SAS1DataCAN3"
  In1/1 -> Bus Selector4/1

== system Control_test/InputProcessing/IBEOCANProcessing/IBEO_ESP2 ==
  Bus Creator : BusCreator  Inputs=12
  ESP2 : rtican/RTICAN Receive (RX)   Reserved1=[]  Reserved2=[]  Reserved3=[]  Reserved4=[]  SfcnMessage=[]  Msg_Struct=[]  BoardTypeNo=[]  BoardNo=[]  ChannelNo=[]  Parameters=[]  DialogFcn=[]  UnitName=[]  Revision=[]  UnitValues=[]  DSProperties=struct('RTI',struct('Version',uint32(5),'BlockType',struct('isSLSource',uint8(1),'isSLSink',uint8(1),'isHWSource',uint8(0),'isHWSink',uint8(0),'isSetup',uint8(0),'isInline',uint8(1),'isNonInline',uint8(0),'isInterrupt',uint8(0),'isChannelwise',uint8(0)),'IOBoardType','RTICAN','UnitType','MESSAGE','Identifier','RX','DialogType','MSVC','BlockSet','RTICAN','SlaveProcessor','CAN'))  RTIBlockInterface=struct('OutputPortsWidth',int32([1 1 1 1 1 1 1 1 1 1 1 1]),'OutputPortsActive',[1 1 1 1 1 1 1 1 1 1 1 1],'OutputPortsName',{{'LAT_ACCEL','LAT_ACCEL_STAT','LAT_ACCEL_DIAG','LONG_ACCEL','LONG_ACCEL_STAT','LONG_ACCEL_DIAG','CYL_PRES','CYL_PRES_STAT','CYL_PRESS_DIAG','YAW_RATE','YAW_RATE_STAT','YAW_RATE_DIAG'}},'OutputPortsDataType',{{'SS_DOUBLE','SS_DOUBLE','SS_DOUBLE','SS_DOUBLE','SS_DOUBLE','SS_DOUBLE','SS_DOUBLE','SS_DOUBLE','SS_DOUBLE','SS_DOUBLE','SS_DOUBLE','SS_DOUBLE'}},'OutputPortsLabel',{{'LAT_ACCEL','LAT_ACCEL_STAT','LAT_ACCEL_DIAG','LONG_ACCEL','LONG_ACCEL_STAT','LONG_ACCEL_DIAG','CYL_PRES','CYL_PRES_STAT','CYL_PRESS_DIAG','YAW_RATE','YAW_RATE_STAT','YAW_RATE_DIAG'}},'OutputPortsLabelMode','ON','InputPortsWidth',int32(0),'InputPortsActive',0,'DialogFcn','rtican_message_interface_gui','BlockDisplay',{{'','center'}},'IconTransparency','on','ParameterTunableNames',{{}},'InitLevel',3,'BlockName',struct('Token',{{'ESP2'}}),'SampleTime',{{-1}},'TriggerPort',{{'none'}},'EnablePort',{{'none'}})  RTIBlockParameters=struct('BoardTypeNo',{{1,'OFF',[]}},'BoardNo',{{2,'ON',[1 16]}},'ChannelNo',{{1,'ON',[1 2]}},'Parameters',{{struct('DataFileSupport',struct('DataFileSelectedMaster',1,'DataFileSelectedLocal',0,'DataFileName','c:\users\mpc_car\documents\github\mpc-car\controller\dbcfiles\ibeo_can_object_and_vehicle_data.dbc|','DataFileDate',['22-10-2012 17:26:29'],'SelectedFile',['<no file selected>'],'InterfaceFcn','rtican_dbc_file_parser'),'Options',struct('StatusSelected',0,'TimeSelected',0,'DeltaTimeSelected',0,'BytePortSelected',0,'MessageLengthSelected',0,'TriggerPort',struct('Selected',0,'TriggerType',0),'UserCoding',struct('Selected',0,'InterfaceFile','UserDecodingFile','FcnName','UserDecodeFcn','InportSelected',0,'InportWidth',1,'OutportSelected',0,'OutportWidth',1),'EnablePortSelected',0,'SignalOnPortnameSelected',1,'UseRXService',0),'Message',struct('MsgOnBlocknameSelected',1,'MsgName','ESP2','MsgIdFormat',0,'MsgId',544,'MsgLength',8,'NumSignals',12,'SampleTime',-1,'Signal',struct('SgnName',{'LAT_ACCEL','LAT_ACCEL_STAT','LAT_ACCEL_DIAG','LONG_ACCEL','LONG_ACCEL_STAT','LONG_ACCEL_DIAG','CYL_PRES','CYL_PRES_STAT','CYL_PRESS_DIAG','YAW_RATE','YAW_RATE_STAT','YAW_RATE_DIAG'},'SgnStartBit',{0,14,15,16,30,31,32,46,47,48,62,63},'SgnLength',{11,1,1,11,1,1,12,1,1,13,1,1},'SgnType',{0,0,0,0,0,0,0,0,0,0,0,0},'ModeValue',{-1,-1,-1,-1,-1,-1,-1,-1,-1,-1,-1,-1},'DataType',{0,0,0,0,0,0,0,0,0,0,0,0},'ByteLayout',{0,0,0,0,0,0,0,0,0,0,0,0},'Factor',{0.01,1,1,0.01,1,1,0.1,1,1,0.01,1,1},'Offset',{-10.23,0,0,-10.23,0,0,0,0,0,-40.95,0,0},'SgnComment',{{''},{''},{''},{''},{''},{''},{''},{''},{''},{''},{''},{''}},'SgnUnit',{'m/s^2','','','m/s^2','','','Bar','','','deg/s','',''},'Min',{-10.23,0,0,-10.23,0,0,0,0,0,-40.95,0,0},'Max',{10.24,1,1,10.24,1,1,409.5,1,1,40.96,1,1},'SLDataType',{'SS_DOUBLE','SS_DOUBLE','SS_DOUBLE','SS_DOUBLE','SS_DOUBLE','SS_DOUBLE','SS_DOUBLE','SS_DOUBLE','SS_DOUBLE','SS_DOUBLE','SS_DOUBLE','SS_DOUBLE'}),'MsgIdNumFormat',0,'MsgComment',{{['[P] Periodic']}}),'Version',1.2,'general',struct('isFromLib',0)),'OFF',[]}},'GroupId',{{struct('Group',{{'RTICAN'}},'No',3,'Behavior',{{'NAMECHANGE'}},'BlockType',{{'SINK'}},'NameChangeFlag',0),'OFF',[]}},'SFcnRTICANMessage',{{struct('MsgType','RX','SFcnPortType','Scalar','MsgName','ESP2','MsgIdFormat','STD','MsgId',544,'MsgLength',8,'NumSignals',12,'SampleTime',-1,'Signal',struct('SgnName',{'LAT_ACCEL','LAT_ACCEL_STAT','LAT_ACCEL_DIAG','LONG_ACCEL','LONG_ACCEL_STAT','LONG_ACCEL_DIAG','CYL_PRES','CYL_PRES_STAT','CYL_PRESS_DIAG','YAW_RATE','YAW_RATE_STAT','YAW_RATE_DIAG'},'SgnStartBit',{0,14,15,16,30,31,32,46,47,48,62,63},'SgnLength',{11,1,1,11,1,1,12,1,1,13,1,1},'SgnType',{'standard','standard','standard','standard','standard','standard','standard','standard','standard','standard','standard','standard'},'ModeValue',{-1,-1,-1,-1,-1,-1,-1,-1,-1,-1,-1,-1},'DataType',{['unsigned int'],['unsigned int'],['unsigned int'],['unsigned int'],['unsigned int'],['unsigned int'],['unsigned int'],['unsigned int'],['unsigned int'],['unsigned int'],['unsigned int'],['unsigned int']},'ByteLayout',{['little endian'],['little endian'],['little endian'],['little endian'],['little endian'],['little endian'],['little endian'],['little endian'],['little endian'],['little endian'],['little endian'],['little endian']},'Factor',{0.01,1,1,0.01,1,1,0.1,1,1,0.01,1,1},'Offset',{-10.23,0,0,-10.23,0,0,0,0,0,-40.95,0,0},'SLDataType',{'SS_DOUBLE','SS_DOUBLE','SS_DOUBLE','SS_DOUBLE','SS_DOUBLE','SS_DOUBLE','SS_DOUBLE','SS_DOUBLE','SS_DOUBLE','SS_DOUBLE','SS_DOUBLE','SS_DOUBLE'}),'StatusSelected','no','TimeSelected','no','DeltaTimeSelected','no','BytePortSelected','no','MessageLengthSelected','no','TriggerPort',struct('Selected','no','TriggerType',0),'UserCoding',struct('Selected','no','InterfaceFile','UserDecodingFile','FcnName','UserDecodeFcn','InportSelected','no','InportWidth',1,'OutportSelected','no','OutportWidth',1),'EnablePortSelected','no','UseRXService','no','BoardType','DS1','BoardNo',2,'ControllerNo',1),'OFF',[]}},'TLCFileName',{{'rtican_rx_message','OFF',[]}})  RTISFcnParameters=struct('SFcnRTICANMessage','struct','TLCFileName','char')  RTIBlockParaDefault=struct('BoardTypeNo',4302,'BoardNo',1,'ChannelNo',1,'Parameters',struct('DataFileSupport',struct('DataFileSelectedMaster',0,'DataFileSelectedLocal',0,'DataFileName','','DataFileDate','','SelectedFile',['<no file selected>']),'Options',struct('StatusSelected',1,'TimeSelected',1,'DeltaTimeSelected',1,'BytePortSelected',0,'MessageLengthSelected',0,'TriggerPort',struct('Selected',0,'TriggerType','rising'),'UserCoding',struct('Selected',0,'InterfaceFile','UserDecodingFile','FcnName','UserDecodeFcn','InportSelected',0,'InportWidth',1,'OutportSelected',0,'OutportWidth',1),'EnablePortSelected',0,'SignalOnPortnameSelected',1,'UseRXService',0),'Message',struct('MsgOnBlocknameSelected',0,'MsgName',['RX Message'],'MsgIdFormat',0,'MsgId',100,'MsgLength',8,'NumSignals',1,'SampleTime',-1,'Signal',struct('SgnName',['RX signal'],'SgnStartBit',0,'SgnLength',8,'SgnType',0,'ModeValue',-1,'DataType',0,'SLDataType','SS_DOUBLE','ByteLayout',0,'Factor',1,'Offset',0,'Min',0,'Max',255,'SgnComment',{{}},'SgnUnit',''),'MsgIdNumFormat',0,'MsgComment',{{''}}),'Version',1.2,'general',struct('isFromLib',1)),'GroupId',struct('Group',{{'RTICAN'}},'No',1,'Behavior',{{'NAMECHANGE'}},'BlockType',{{'SINK'}},'NameChangeFlag',0),'SFcnRTICANMessage',struct('MsgType','RX','MsgName',['RX Message'],'MsgIdFormat','STD','MsgId',100,'MsgLength',8,'NumSignals',1,'SampleTime',-1,'Signal',struct('SgnName',['RX signal'],'SgnStartBit',0,'SgnLength',8,'SgnType','standard','ModeValue',-1,'DataType',['unsigned int'],'ByteLayout',['little endian'],'SLDataType','SS_DOUBLE','Factor',1,'Offset',0),'StatusSelected','yes','TimeSelected','yes','DeltaTimeSelected','yes','BytePortSelected','no','MessageLengthSelected','no','EnablePortSelected','no','UserCoding',struct('Selected','no','InterfaceFile','UserDecodingFile','FcnName','UserDecodeFcn','InportSelected','no','InportWidth',1,'OutportSelected','no','OutportWidth',1),'TriggerPort',struct('Selected','no','TriggerType','rising'),'UseRXService','no','BoardType','DS4302','BoardNo',1,'ControllerNo',1,'SFcnPortType','Scalar'),'TLCFileName','rtican_rx_message')
      settings: AttributesFormatString=Group Id: RTICAN3\n
  ESP2_CAN : Outport
  wires:
  Bus Creator/1 -> ESP2_CAN/1  "ESP2_CAN"
  ESP2/1 -> Bus Creator/1  "LAT_ACCEL"
  ESP2/2 -> Bus Creator/2  "LAT_ACCEL_STAT"
  ESP2/3 -> Bus Creator/3  "LAT_ACCEL_DIAG"
  ESP2/4 -> Bus Creator/4  "LONG_ACCEL"
  ESP2/5 -> Bus Creator/5  "LONG_ACCEL_STAT"
  ESP2/6 -> Bus Creator/6  "LONG_ACCEL_DIAG"
  ESP2/7 -> Bus Creator/7  "CYL_PRES"
  ESP2/8 -> Bus Creator/8  "CYL_PRES_STAT"
  ESP2/9 -> Bus Creator/9  "CYL_PRESS_DIAG"
  ESP2/10 -> Bus Creator/10  "YAW_RATE"
  ESP2/11 -> Bus Creator/11  "YAW_RATE_STAT"
  ESP2/12 -> Bus Creator/12  "YAW_RATE_DIAG"

== system Control_test/InputProcessing/IBEOCANProcessing/IBEO_SAS1 ==
  Bus Creator : BusCreator  Inputs=5
  SAS11 : rtican/RTICAN Receive (RX)   Reserved1=[]  Reserved2=[]  Reserved3=[]  Reserved4=[]  SfcnMessage=[]  Msg_Struct=[]  BoardTypeNo=[]  BoardNo=[]  ChannelNo=[]  Parameters=[]  DialogFcn=[]  UnitName=[]  Revision=[]  UnitValues=[]  DSProperties=struct('RTI',struct('Version',uint32(5),'BlockType',struct('isSLSource',uint8(1),'isSLSink',uint8(1),'isHWSource',uint8(0),'isHWSink',uint8(0),'isSetup',uint8(0),'isInline',uint8(1),'isNonInline',uint8(0),'isInterrupt',uint8(0),'isChannelwise',uint8(0)),'IOBoardType','RTICAN','UnitType','MESSAGE','Identifier','RX','DialogType','MSVC','BlockSet','RTICAN','SlaveProcessor','CAN'))  RTIBlockInterface=struct('OutputPortsWidth',int32([1 1 1 1 1]),'OutputPortsActive',[1 1 1 1 1],'OutputPortsName',{{'SAS_Angle','SAS_Speed','SAS_Stat','MsgCount','CheckSum'}},'OutputPortsDataType',{{'SS_DOUBLE','SS_DOUBLE','SS_DOUBLE','SS_DOUBLE','SS_DOUBLE'}},'OutputPortsLabel',{{'SAS_Angle','SAS_Speed','SAS_Stat','MsgCount','CheckSum'}},'OutputPortsLabelMode','ON','InputPortsWidth',int32(0),'InputPortsActive',0,'DialogFcn','rtican_message_interface_gui','BlockDisplay',{{'','center'}},'IconTransparency','on','ParameterTunableNames',{{}},'InitLevel',3,'BlockName',struct('Token',{{'SAS1'}}),'SampleTime',{{-1}},'TriggerPort',{{'none'}},'EnablePort',{{'none'}})  RTIBlockParameters=struct('BoardTypeNo',{{1,'OFF',[]}},'BoardNo',{{2,'ON',[1 16]}},'ChannelNo',{{1,'ON',[1 2]}},'Parameters',{{struct('DataFileSupport',struct('DataFileSelectedMaster',1,'DataFileSelectedLocal',0,'DataFileName','c:\users\mpc_car\documents\github\mpc-car\controller\dbcfiles\ibeo_can_object_and_vehicle_data.dbc|','DataFileDate',['22-10-2012 17:26:29'],'SelectedFile',['<no file selected>'],'InterfaceFcn','rtican_dbc_file_parser'),'Options',struct('StatusSelected',0,'TimeSelected',0,'DeltaTimeSelected',0,'BytePortSelected',0,'MessageLengthSelected',0,'TriggerPort',struct('Selected',0,'TriggerType',0),'UserCoding',struct('Selected',0,'InterfaceFile','UserDecodingFile','FcnName','UserDecodeFcn','InportSelected',0,'InportWidth',1,'OutportSelected',0,'OutportWidth',1),'EnablePortSelected',0,'SignalOnPortnameSelected',1,'UseRXService',0),'Message',struct('MsgOnBlocknameSelected',1,'MsgName','SAS1','MsgIdFormat',0,'MsgId',688,'MsgLength',5,'NumSignals',5,'SampleTime',-1,'Signal',struct('SgnName',{'SAS_Angle','SAS_Speed','SAS_Stat','MsgCount','CheckSum'},'SgnStartBit',{0,16,24,32,36},'SgnLength',{16,8,8,4,4},'SgnType',{0,0,0,0,0},'ModeValue',{-1,-1,-1,-1,-1},'DataType',{0,0,0,0,0},'ByteLayout',{0,0,0,0,0},'Factor',{0.1,4,1,1,1},'Offset',{0,0,0,0,0},'SgnComment',{{['When MDPS ECU sends this message, this message value is valid 1.5 sec later from IG-ON.']},{['When MDPS ECU sends this message, this message value is valid 1.5 sec later from IG-ON.']},{['When MDPS ECU sends this message, this message value is valid 1.5 sec later from IG-ON.']},{['When MDPS ECU sends this message, this message value is valid 1.5 sec later from IG-ON.']},{['When MDPS ECU sends this message, this message value is valid 1.5 sec later from IG-ON.']}},'SgnUnit',{'Deg','','','',''},'Min',{-3276.8,0,0,0,0},'Max',{3276.7,1016,255,15,15},'SLDataType',{'SS_DOUBLE','SS_DOUBLE','SS_DOUBLE','SS_DOUBLE','SS_DOUBLE'}),'MsgIdNumFormat',1,'MsgComment',{{['[P] Periodic']}}),'Version',1.2,'general',struct('isFromLib',0)),'OFF',[]}},'GroupId',{{struct('Group',{{'RTICAN'}},'No',3,'Behavior',{{'NAMECHANGE'}},'BlockType',{{'SINK'}},'NameChangeFlag',0),'OFF',[]}},'SFcnRTICANMessage',{{struct('MsgType','RX','SFcnPortType','Scalar','MsgName','SAS1','MsgIdFormat','STD','MsgId',688,'MsgLength',5,'NumSignals',5,'SampleTime',-1,'Signal',struct('SgnName',{'SAS_Angle','SAS_Speed','SAS_Stat','MsgCount','CheckSum'},'SgnStartBit',{0,16,24,32,36},'SgnLength',{16,8,8,4,4},'SgnType',{'standard','standard','standard','standard','standard'},'ModeValue',{-1,-1,-1,-1,-1},'DataType',{['unsigned int'],['unsigned int'],['unsigned int'],['unsigned int'],['unsigned int']},'ByteLayout',{['little endian'],['little endian'],['little endian'],['little endian'],['little endian']},'Factor',{0.1,4,1,1,1},'Offset',{0,0,0,0,0},'SLDataType',{'SS_DOUBLE','SS_DOUBLE','SS_DOUBLE','SS_DOUBLE','SS_DOUBLE'}),'StatusSelected','no','TimeSelected','no','DeltaTimeSelected','no','BytePortSelected','no','MessageLengthSelected','no','TriggerPort',struct('Selected','no','TriggerType',0),'UserCoding',struct('Selected','no','InterfaceFile','UserDecodingFile','FcnName','UserDecodeFcn','InportSelected','no','InportWidth',1,'OutportSelected','no','OutportWidth',1),'EnablePortSelected','no','UseRXService','no','BoardType','DS1','BoardNo',2,'ControllerNo',1),'OFF',[]}},'TLCFileName',{{'rtican_rx_message','OFF',[]}})  RTISFcnParameters=struct('SFcnRTICANMessage','struct','TLCFileName','char')  RTIBlockParaDefault=struct('BoardTypeNo',4302,'BoardNo',1,'ChannelNo',1,'Parameters',struct('DataFileSupport',struct('DataFileSelectedMaster',0,'DataFileSelectedLocal',0,'DataFileName','','DataFileDate','','SelectedFile',['<no file selected>']),'Options',struct('StatusSelected',1,'TimeSelected',1,'DeltaTimeSelected',1,'BytePortSelected',0,'MessageLengthSelected',0,'TriggerPort',struct('Selected',0,'TriggerType','rising'),'UserCoding',struct('Selected',0,'InterfaceFile','UserDecodingFile','FcnName','UserDecodeFcn','InportSelected',0,'InportWidth',1,'OutportSelected',0,'OutportWidth',1),'EnablePortSelected',0,'SignalOnPortnameSelected',1,'UseRXService',0),'Message',struct('MsgOnBlocknameSelected',0,'MsgName',['RX Message'],'MsgIdFormat',0,'MsgId',100,'MsgLength',8,'NumSignals',1,'SampleTime',-1,'Signal',struct('SgnName',['RX signal'],'SgnStartBit',0,'SgnLength',8,'SgnType',0,'ModeValue',-1,'DataType',0,'SLDataType','SS_DOUBLE','ByteLayout',0,'Factor',1,'Offset',0,'Min',0,'Max',255,'SgnComment',{{}},'SgnUnit',''),'MsgIdNumFormat',0,'MsgComment',{{''}}),'Version',1.2,'general',struct('isFromLib',1)),'GroupId',struct('Group',{{'RTICAN'}},'No',1,'Behavior',{{'NAMECHANGE'}},'BlockType',{{'SINK'}},'NameChangeFlag',0),'SFcnRTICANMessage',struct('MsgType','RX','MsgName',['RX Message'],'MsgIdFormat','STD','MsgId',100,'MsgLength',8,'NumSignals',1,'SampleTime',-1,'Signal',struct('SgnName',['RX signal'],'SgnStartBit',0,'SgnLength',8,'SgnType','standard','ModeValue',-1,'DataType',['unsigned int'],'ByteLayout',['little endian'],'SLDataType','SS_DOUBLE','Factor',1,'Offset',0),'StatusSelected','yes','TimeSelected','yes','DeltaTimeSelected','yes','BytePortSelected','no','MessageLengthSelected','no','EnablePortSelected','no','UserCoding',struct('Selected','no','InterfaceFile','UserDecodingFile','FcnName','UserDecodeFcn','InportSelected','no','InportWidth',1,'OutportSelected','no','OutportWidth',1),'TriggerPort',struct('Selected','no','TriggerType','rising'),'UseRXService','no','BoardType','DS4302','BoardNo',1,'ControllerNo',1,'SFcnPortType','Scalar'),'TLCFileName','rtican_rx_message')
      settings: AttributesFormatString=Group Id: RTICAN3\n
  SAS1_CAN : Outport
  wires:
  Bus Creator/1 -> SAS1_CAN/1  "SAS1_CAN"
  SAS11/1 -> Bus Creator/1  "SAS_Angle"
  SAS11/2 -> Bus Creator/2  "SAS_Speed"
  SAS11/3 -> Bus Creator/3  "SAS_Stat"
  SAS11/4 -> Bus Creator/4  "MsgCount"
  SAS11/5 -> Bus Creator/5  "CheckSum"
